simulink model "fdatool4"  (Simulink 5.1)
settings: Solver=ode45  StartTime=0.0  StopTime=0.5  RelTol=1e-3
libraries: fixpt_lib_4 x10, dspsigops x7
settings Model: Creator=svenhoffmann  LastModifiedBy=svenhoffmann  ExtModeAutoUpdateStatusClock=off  BooleanDataType=on  ProdHWDeviceType=Microprocessor

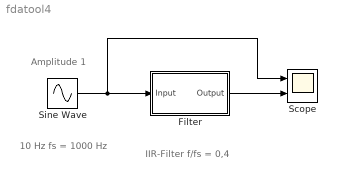
== system fdatool4 ==
  note: Amplitude 1
  note: 10 Hz
      | fs = 1000 Hz
  note: IIR-Filter
      | f/fs = 0,4
  Filter : Subsystem  Tag=FilterWizardSubSystem
  Scope : Scope  NumInputPorts=2
      settings: YMin=-5~-5  YMax=5~5
  Sine Wave : Sin  Amplitude=0.99996948  Frequency=2*pi*10  SampleTime=1/1000
  wires:
  Sine Wave/1 -> Filter/1(Input), Scope/1
  Filter/1(Output) -> Scope/2

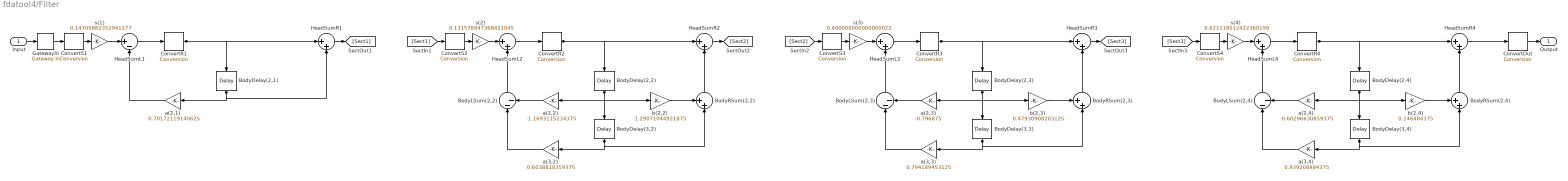
== system fdatool4/Filter ==
  Input : Inport
  BodyDelay(2,1) : dspsigops/Delay  Orientation=down  dly_unit=Samples  delay=1  ic_detail=off  dif_ic_for_ch=off  dif_ic_for_dly=off  ic=0  reset_popup=None
  BodyDelay(2,2) : dspsigops/Delay  Orientation=down  dly_unit=Samples  delay=1  ic_detail=off  dif_ic_for_ch=off  dif_ic_for_dly=off  ic=0  reset_popup=None
  BodyDelay(2,3) : dspsigops/Delay  Orientation=down  dly_unit=Samples  delay=1  ic_detail=off  dif_ic_for_ch=off  dif_ic_for_dly=off  ic=0  reset_popup=None
  BodyDelay(2,4) : dspsigops/Delay  Orientation=down  dly_unit=Samples  delay=1  ic_detail=off  dif_ic_for_ch=off  dif_ic_for_dly=off  ic=0  reset_popup=None
  BodyDelay(3,2) : dspsigops/Delay  Orientation=down  dly_unit=Samples  delay=1  ic_detail=off  dif_ic_for_ch=off  dif_ic_for_dly=off  ic=0  reset_popup=None
  BodyDelay(3,3) : dspsigops/Delay  Orientation=down  dly_unit=Samples  delay=1  ic_detail=off  dif_ic_for_ch=off  dif_ic_for_dly=off  ic=0  reset_popup=None
  BodyDelay(3,4) : dspsigops/Delay  Orientation=down  dly_unit=Samples  delay=1  ic_detail=off  dif_ic_for_ch=off  dif_ic_for_dly=off  ic=0  reset_popup=None
  BodyLSum(2,2) : Sum  Orientation=up  Inputs=|--  ShowAdditionalParam=on  OutDataTypeMode=Specify via dialog  OutDataType=sfix(32)  OutScaling=2^-30  SaturateOnIntegerOverflow=on  LockScale=on
  BodyLSum(2,3) : Sum  Orientation=up  Inputs=|--  ShowAdditionalParam=on  OutDataTypeMode=Specify via dialog  OutDataType=sfix(32)  OutScaling=2^-30  SaturateOnIntegerOverflow=on  LockScale=on
  BodyLSum(2,4) : Sum  Orientation=up  Inputs=|--  ShowAdditionalParam=on  OutDataTypeMode=Specify via dialog  OutDataType=sfix(32)  OutScaling=2^-30  SaturateOnIntegerOverflow=on  LockScale=on
  BodyRSum(2,2) : Sum  Orientation=up  Inputs=++|  ShowAdditionalParam=on  OutDataTypeMode=Specify via dialog  OutDataType=sfix(32)  OutScaling=2^-30  SaturateOnIntegerOverflow=on  LockScale=on
  BodyRSum(2,3) : Sum  Orientation=up  Inputs=++|  ShowAdditionalParam=on  OutDataTypeMode=Specify via dialog  OutDataType=sfix(32)  OutScaling=2^-30  SaturateOnIntegerOverflow=on  LockScale=on
  BodyRSum(2,4) : Sum  Orientation=up  Inputs=++|  ShowAdditionalParam=on  OutDataTypeMode=Specify via dialog  OutDataType=sfix(32)  OutScaling=2^-30  SaturateOnIntegerOverflow=on  LockScale=on
  ConvertOut : fixpt_lib_4/Data Type/Conversion  ConvertRealWorld=Real World Value  OutputDataTypeScalingMode=Specify via dialog  OutDataType=sfix(16)  OutScaling=2^-15  DoSatur=on
      settings: LockScale=on
  ConvertR{1..4} (4 alike) : fixpt_lib_4/Data Type/Conversion  ConvertRealWorld=Real World Value  OutputDataTypeScalingMode=Specify via dialog  OutDataType=sfix(16)  OutScaling=2^-15  DoSatur=on
      settings: LockScale=on
  ConvertS{1..4} (4 alike) : fixpt_lib_4/Data Type/Conversion  ConvertRealWorld=Real World Value  OutputDataTypeScalingMode=Specify via dialog  OutDataType=sfix(16)  OutScaling=2^-15  DoSatur=on
      settings: LockScale=on
  GatewayIn : fixpt_lib_4/Data Type/Gateway In  InRealWorld=Real World Value  OutputDataTypeScalingMode=Specify via dialog  OutDataType=sfix(16)  OutScaling=2^-15  DoSatur=on
      settings: LockScale=on
  HeadSumL1 : Sum  Inputs=|+-  ShowAdditionalParam=on  OutDataTypeMode=Specify via dialog  OutDataType=sfix(32)  OutScaling=2^-30  SaturateOnIntegerOverflow=on  LockScale=on
  HeadSumL2 : Sum  Inputs=|++  ShowAdditionalParam=on  OutDataTypeMode=Specify via dialog  OutDataType=sfix(32)  OutScaling=2^-30  SaturateOnIntegerOverflow=on  LockScale=on
  HeadSumL3 : Sum  Inputs=|++  ShowAdditionalParam=on  OutDataTypeMode=Specify via dialog  OutDataType=sfix(32)  OutScaling=2^-30  SaturateOnIntegerOverflow=on  LockScale=on
  HeadSumL4 : Sum  Inputs=|++  ShowAdditionalParam=on  OutDataTypeMode=Specify via dialog  OutDataType=sfix(32)  OutScaling=2^-30  SaturateOnIntegerOverflow=on  LockScale=on
  HeadSumR{1..4} (4 alike) : Sum  Inputs=|++  ShowAdditionalParam=on  OutDataTypeMode=Specify via dialog  OutDataType=sfix(32)  OutScaling=2^-30  SaturateOnIntegerOverflow=on  LockScale=on
  a(2,1) : Gain  Orientation=left  Gain=-0.70172119140625  ShowAdditionalParam=on  ParameterDataTypeMode=Specify via dialog  ParameterScalingMode=Use specified scaling  ParameterScaling=2^-14  OutDataTypeMode=Specify via dialog  OutDataType=sfix(32)  OutScaling=2^-30  SaturateOnIntegerOverflow=on  LockScale=on
  a(2,2) : Gain  Orientation=left  Gain=-1.1693115234375  ShowAdditionalParam=on  ParameterDataTypeMode=Specify via dialog  ParameterScalingMode=Use specified scaling  ParameterScaling=2^-14  OutDataTypeMode=Specify via dialog  OutDataType=sfix(32)  OutScaling=2^-30  SaturateOnIntegerOverflow=on  LockScale=on
  a(2,3) : Gain  Orientation=left  Gain=-0.796875  ShowAdditionalParam=on  ParameterDataTypeMode=Specify via dialog  ParameterScalingMode=Use specified scaling  ParameterScaling=2^-14  OutDataTypeMode=Specify via dialog  OutDataType=sfix(32)  OutScaling=2^-30  SaturateOnIntegerOverflow=on  LockScale=on
  a(2,4) : Gain  Orientation=left  Gain=-0.60296630859375  ShowAdditionalParam=on  ParameterDataTypeMode=Specify via dialog  ParameterScalingMode=Use specified scaling  ParameterScaling=2^-14  OutDataTypeMode=Specify via dialog  OutDataType=sfix(32)  OutScaling=2^-30  SaturateOnIntegerOverflow=on  LockScale=on
  a(3,2) : Gain  Orientation=left  Gain=0.6038818359375  ShowAdditionalParam=on  ParameterDataTypeMode=Specify via dialog  ParameterScalingMode=Use specified scaling  ParameterScaling=2^-14  OutDataTypeMode=Specify via dialog  OutDataType=sfix(32)  OutScaling=2^-30  SaturateOnIntegerOverflow=on  LockScale=on
  a(3,3) : Gain  Orientation=left  Gain=0.794189453125  ShowAdditionalParam=on  ParameterDataTypeMode=Specify via dialog  ParameterScalingMode=Use specified scaling  ParameterScaling=2^-14  OutDataTypeMode=Specify via dialog  OutDataType=sfix(32)  OutScaling=2^-30  SaturateOnIntegerOverflow=on  LockScale=on
  a(3,4) : Gain  Orientation=left  Gain=0.939208984375  ShowAdditionalParam=on  ParameterDataTypeMode=Specify via dialog  ParameterScalingMode=Use specified scaling  ParameterScaling=2^-14  OutDataTypeMode=Specify via dialog  OutDataType=sfix(32)  OutScaling=2^-30  SaturateOnIntegerOverflow=on  LockScale=on
  b(2,2) : Gain  Gain=1.29071044921875  ShowAdditionalParam=on  ParameterDataTypeMode=Specify via dialog  ParameterScalingMode=Use specified scaling  ParameterScaling=2^-14  OutDataTypeMode=Specify via dialog  OutDataType=sfix(32)  OutScaling=2^-30  SaturateOnIntegerOverflow=on  LockScale=on
  b(2,3) : Gain  Gain=0.47930908203125  ShowAdditionalParam=on  ParameterDataTypeMode=Specify via dialog  ParameterScalingMode=Use specified scaling  ParameterScaling=2^-14  OutDataTypeMode=Specify via dialog  OutDataType=sfix(32)  OutScaling=2^-30  SaturateOnIntegerOverflow=on  LockScale=on
  b(2,4) : Gain  Gain=0.146484375  ShowAdditionalParam=on  ParameterDataTypeMode=Specify via dialog  ParameterScalingMode=Use specified scaling  ParameterScaling=2^-14  OutDataTypeMode=Specify via dialog  OutDataType=sfix(32)  OutScaling=2^-30  SaturateOnIntegerOverflow=on  LockScale=on
  s(1) : Gain  Gain=0.14705882352941177  ShowAdditionalParam=on  ParameterDataTypeMode=Specify via dialog  ParameterScalingMode=Use specified scaling  ParameterScaling=2^-14  OutDataTypeMode=Specify via dialog  OutDataType=sfix(32)  OutScaling=2^-30  SaturateOnIntegerOverflow=on  LockScale=on
  s(2) : Gain  Gain=0.131578947368421045  ShowAdditionalParam=on  ParameterDataTypeMode=Specify via dialog  ParameterScalingMode=Use specified scaling  ParameterScaling=2^-14  OutDataTypeMode=Specify via dialog  OutDataType=sfix(32)  OutScaling=2^-30  SaturateOnIntegerOverflow=on  LockScale=on
  s(3) : Gain  Gain=0.400000000000000022  ShowAdditionalParam=on  ParameterDataTypeMode=Specify via dialog  ParameterScalingMode=Use specified scaling  ParameterScaling=2^-14  OutDataTypeMode=Specify via dialog  OutDataType=sfix(32)  OutScaling=2^-30  SaturateOnIntegerOverflow=on  LockScale=on
  s(4) : Gain  Gain=0.621118012422360199  ShowAdditionalParam=on  ParameterDataTypeMode=Specify via dialog  ParameterScalingMode=Use specified scaling  ParameterScaling=2^-14  OutDataTypeMode=Specify via dialog  OutDataType=sfix(32)  OutScaling=2^-30  SaturateOnIntegerOverflow=on  LockScale=on
  Output : Outport
  wires:
  s(1)/1 -> HeadSumL1/1
  HeadSumR1/1 -> [Sect1]
  BodyDelay(2,1)/1 -> a(2,1)/1, HeadSumR1/2
  a(2,1)/1 -> HeadSumL1/2
  s(2)/1 -> HeadSumL2/1
  HeadSumR2/1 -> [Sect2]
  BodyDelay(2,2)/1 -> a(2,2)/1, b(2,2)/1, BodyDelay(3,2)/1
  a(2,2)/1 -> BodyLSum(2,2)/2
  b(2,2)/1 -> BodyRSum(2,2)/1
  BodyLSum(2,2)/1 -> HeadSumL2/2
  BodyRSum(2,2)/1 -> HeadSumR2/2
  BodyDelay(3,2)/1 -> a(3,2)/1, BodyRSum(2,2)/2
  a(3,2)/1 -> BodyLSum(2,2)/1
  s(3)/1 -> HeadSumL3/1
  HeadSumR3/1 -> [Sect3]
  BodyDelay(2,3)/1 -> a(2,3)/1, b(2,3)/1, BodyDelay(3,3)/1
  a(2,3)/1 -> BodyLSum(2,3)/2
  b(2,3)/1 -> BodyRSum(2,3)/1
  BodyLSum(2,3)/1 -> HeadSumL3/2
  BodyRSum(2,3)/1 -> HeadSumR3/2
  BodyDelay(3,3)/1 -> a(3,3)/1, BodyRSum(2,3)/2
  a(3,3)/1 -> BodyLSum(2,3)/1
  s(4)/1 -> HeadSumL4/1
  BodyDelay(2,4)/1 -> a(2,4)/1, b(2,4)/1, BodyDelay(3,4)/1
  a(2,4)/1 -> BodyLSum(2,4)/2
  b(2,4)/1 -> BodyRSum(2,4)/1
  BodyLSum(2,4)/1 -> HeadSumL4/2
  BodyRSum(2,4)/1 -> HeadSumR4/2
  BodyDelay(3,4)/1 -> a(3,4)/1, BodyRSum(2,4)/2
  a(3,4)/1 -> BodyLSum(2,4)/1
  ConvertS1/1 -> s(1)/1
  [Sect1] -> ConvertS2/1
  ConvertS2/1 -> s(2)/1
  [Sect2] -> ConvertS3/1
  ConvertS3/1 -> s(3)/1
  [Sect3] -> ConvertS4/1
  ConvertS4/1 -> s(4)/1
  HeadSumL1/1 -> ConvertR1/1
  ConvertR1/1 -> HeadSumR1/1, BodyDelay(2,1)/1
  HeadSumL2/1 -> ConvertR2/1
  ConvertR2/1 -> HeadSumR2/1, BodyDelay(2,2)/1
  HeadSumL3/1 -> ConvertR3/1
  ConvertR3/1 -> HeadSumR3/1, BodyDelay(2,3)/1
  HeadSumL4/1 -> ConvertR4/1
  ConvertR4/1 -> HeadSumR4/1, BodyDelay(2,4)/1
  HeadSumR4/1 -> ConvertOut/1
  ConvertOut/1 -> Output/1
  Input/1 -> GatewayIn/1
  GatewayIn/1 -> ConvertS1/1
